simulink model "Gesamtmodell_Test"  (R2020a)
settings: Solver=VariableStepAuto  StartTime=0.0  StopTime=30  MaxStep=0.01  RelTol=1e-3
Description:
  | Modell des Gleichstrommotors
  | Eingang: Spannung
  | Ausgang: Kraft
settings Model: Creator=Tobias  LastModifiedBy=Tobias

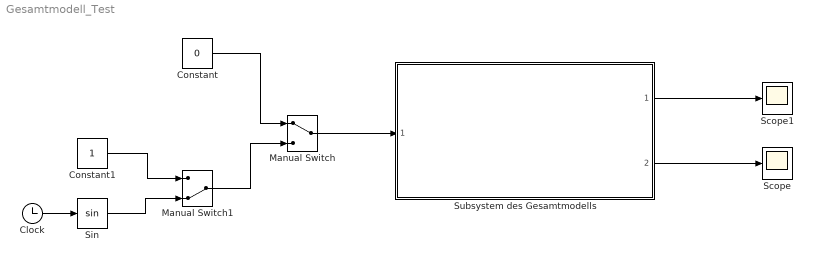
== system Gesamtmodell_Test ==
  Clock : Clock
  Constant : Constant  Value=0
  Constant1 : Constant
  Manual Switch : ManualSwitch
  Manual Switch1 : ManualSwitch  CurrentSetting=0
  Scope : Scope
  Scope1 : Scope
  Sin : Trigonometry
  Subsystem des Gesamtmodells : Subsystem  ReferencedSubsystem=Gesamtmodell  ModellParameter=simparams.gesamtmodell
  wires:
  Constant/1 -> Manual Switch/1
  Subsystem des Gesamtmodells/2 -> Scope/1
  Subsystem des Gesamtmodells/1 -> Scope1/1
  Manual Switch/1 -> Subsystem des Gesamtmodells/1
  Manual Switch1/1 -> Manual Switch/2
  Constant1/1 -> Manual Switch1/1
  Sin/1 -> Manual Switch1/2
  Clock/1 -> Sin/1
